simulink model "zad4_sim"  (R2022b)
settings: Solver=VariableStepAuto  StartTime=0.0  StopTime=10.0  RelTol=1e-3
values from neighbouring files (symbols this model uses):
  l1 = L(1)    [zad4.m]
  l2 = L(2)    [zad4.m]
  l3 = L(3)    [zad4.m]
settings Model: Creator=Mat  LastModifiedBy=Mat

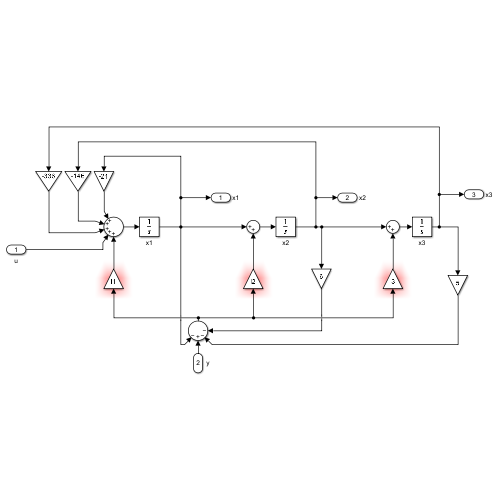
[thumbnail: Simulink's stored preview of the top-level diagram]
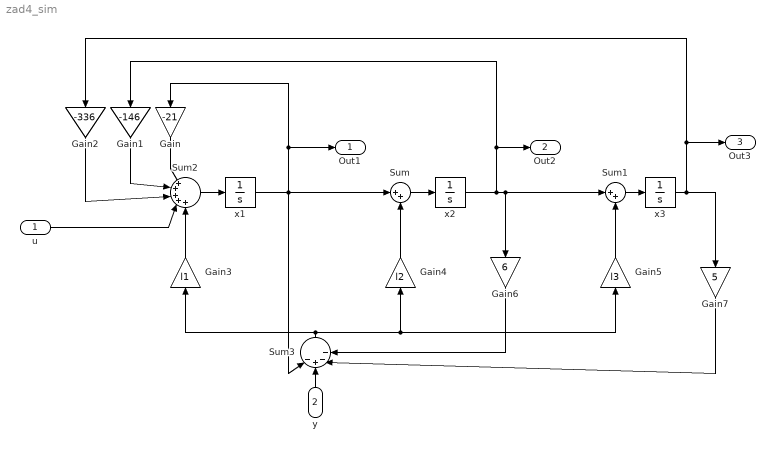
== system zad4_sim ==
  u : Inport
  y : Inport  Port=2
  Gain : Gain  Gain=-21
  Gain1 : Gain  Gain=-146
  Gain2 : Gain  Gain=-336
  Gain3 : Gain  Gain=l1
  Gain4 : Gain  Gain=l2
  Gain5 : Gain  Gain=l3
  Gain6 : Gain  Gain=6
  Gain7 : Gain  Gain=5
  Sum : Sum  Inputs=|++
  Sum1 : Sum  Inputs=|++
  Sum2 : Sum  Inputs=|+++++
  Sum3 : Sum  Inputs=|-+--
  x1 : Integrator
  x2 : Integrator
  x3 : Integrator
  Out1 : Outport  SignalName=x1
  Out2 : Outport  Port=2  SignalName=x2
  Out3 : Outport  Port=3  SignalName=x3
  wires:
  Sum2/1 -> x1/1
  Sum/1 -> x2/1
  x1/1 -> Sum3/1, Out1/1, Gain/1, Sum/1
  Gain/1 -> Sum2/1
  Sum1/1 -> x3/1
  x2/1 -> Gain6/1, Sum1/1, Out2/1, Gain1/1
  x3/1 -> Gain7/1, Out3/1, Gain2/1
  Gain1/1 -> Sum2/2
  Gain2/1 -> Sum2/3
  u/1 -> Sum2/4
  Gain3/1 -> Sum2/5
  Gain4/1 -> Sum/2
  Gain5/1 -> Sum1/2
  y/1 -> Sum3/2
  Sum3/1 -> Gain4/1, Gain5/1, Gain3/1
  Gain6/1 -> Sum3/4
  Gain7/1 -> Sum3/3
